simulink library "drivecyclelib"  (R2016a)
settings: Solver=ode45  StartTime=0.0  StopTime=10.0  RelTol=1e-3
undefined symbols (not defined in the file or in its folder): S_CYCLE, T_CYCLE, T_MAX
libraries: simulink x2
settings Model: Creator=e102261  LastModifiedBy=e102261
settings DataIOCC: LimitDataPoints=on  SaveFormat=Array
settings OptimizationCC: ExpressionDepthLimit=2147483647
settings DebuggingCC: UnderspecifiedInitializationDetection=Classic  MergeDetectMultiDrivingBlocksExec=none  SolverPrmCheckMsg=warning  MultiTaskDSMMsg=warning  MultiTaskCondExecSysMsg=none  FcnCallInpInsideContextMsg=EnableAllAsWarning  StateNameClashWarn=warning  StrictBusMsg=None
settings HardwareCC: ProdBitPerPointer=32  ProdLargestAtomicFloat=None  ProdIntDivRoundTo=Undefined  ProdEndianess=Unspecified  ProdWordSize=32  ProdHWDeviceType=32-bit Generic
settings ModelReferenceCC: PropagateSignalLabelsOutOfModel=off

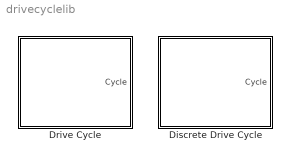
== system drivecyclelib ==
  Discrete Drive Cycle : Subsystem  mask(Discrete Drive Cycle){CycleName=NEDC, CycleRepeatsForever=off, SampleTime=0.1}
      mask prompts: CycleName "Cycle name:"; CycleRepeatsForever "Repeat cycle forever"; SampleTime "Sample time:"
      mask help: This block produces drive cycle data, as used in many automotive applications. It outputs displacement, velocity and acceleration, all in SI units. The user can choose from a list of popular cycles. Accuracy will suffer if the sample time gets too big: the maximum 'safe' value is one.
      mask init:
      | [S_CYCLE, T_CYCLE, T_MAX, W_SCALE, Disp, Vel, Acc, t, v] = ...
      |     drivecyclelib_maskInitFcn(CycleName, CycleRepeatsForever);
      mask TypeOptions CycleName: NEDC | ECE R15 | EUDC | ArtUrban | ArtRoad | ArtMw130 | ArtMw150 | WLTP class 3 | UDDS | FTP | HWFET
      mask Display:
      | color('yellow')
      | plot(t/max(t),3.6*v/160);
      | color('blue')
      | fprintf(CycleName);
  Drive Cycle : Subsystem  mask(Drive Cycle){CycleName=WLTP class 3, CycleRepeatsForever=off}
      mask prompts: CycleName "Cycle name:"; CycleRepeatsForever "Repeat cycle forever"
      mask help: This block produces drive cycle data, as used in many automotive applications. It outputs displacement, velocity and acceleration, all in SI units. The user can choose from a list of popular cycles.
      mask init:
      | [S_CYCLE, T_CYCLE, T_MAX, W_SCALE, Disp, Vel, Acc, t, v] = ...
      |     drivecyclelib_maskInitFcn(CycleName, CycleRepeatsForever);
      mask TypeOptions CycleName: NEDC | ECE R15 | EUDC | ArtUrban | ArtRoad | ArtMw130 | ArtMw150 | WLTP class 3 | UDDS | FTP | HWFET
      mask Display:
      | color('yellow')
      | plot(t/max(t),3.6*v/160);
      | color('blue')
      | fprintf(CycleName);

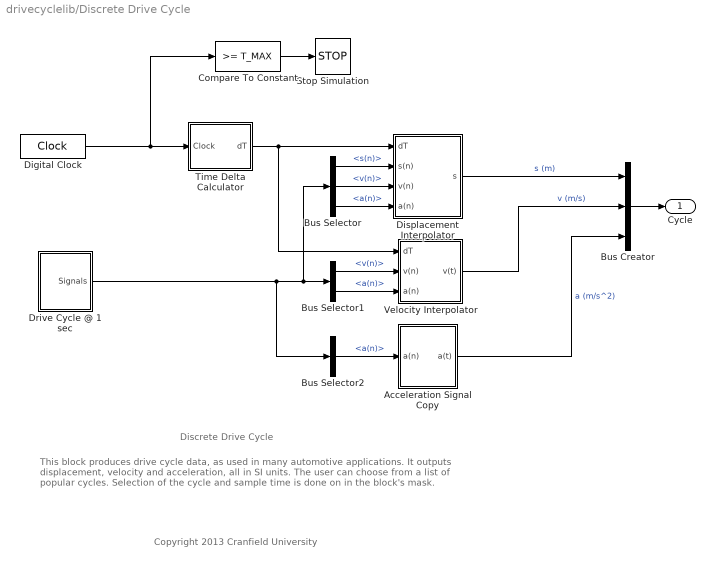
== system drivecyclelib/Discrete Drive Cycle ==
  note: This block produces drive cycle data, as used in many automotive applications.  It outputs
      | displacement, velocity and acceleration, all in SI units.  The user can choose from a list of
      | popular cycles.
      |
      | Selection of the cycle and sample time is done on in the block's mask.
  note: Copyright 2013 Cranfield University
  note: Discrete Drive Cycle
  Acceleration Signal Copy : Subsystem
  Bus Creator : BusCreator  Inputs=3
  Bus Selector : BusSelector  OutputSignals=s(n),v(n),a(n)
  Bus Selector1 : BusSelector  OutputSignals=v(n),a(n)
  Bus Selector2 : BusSelector  OutputSignals=a(n)
  Compare To Constant : simulink/Logic and Bit Operations/Compare To Constant  relop=>=  const=T_MAX  OutDataTypeStr=boolean
  Digital Clock : DigitalClock  SampleTime=SampleTime
  Displacement Interpolator : Subsystem
  Drive Cycle @ 1 sec : Subsystem
  Stop Simulation : Stop
  Time Delta Calculator : Subsystem
  Velocity Interpolator : Subsystem
  Cycle : Outport  SampleTime=SampleTime
  wires:
  Compare To Constant/1 -> Stop Simulation/1
  Time Delta Calculator/1(dT) -> Displacement Interpolator/1(dT), Velocity Interpolator/1(dT)
  Displacement Interpolator/1(s) -> Bus Creator/1  "s (m)"
  Velocity Interpolator/1(v(t)) -> Bus Creator/2  "v (m/s)"
  Drive Cycle @ 1 sec/1(Signals) -> Bus Selector/1, Bus Selector1/1, Bus Selector2/1
  Bus Selector/1 -> Displacement Interpolator/2(s(n))  "<s(n)>"
  Bus Selector/2 -> Displacement Interpolator/3(v(n))  "<v(n)>"
  Bus Selector/3 -> Displacement Interpolator/4(a(n))  "<a(n)>"
  Bus Selector1/1 -> Velocity Interpolator/2(v(n))  "<v(n)>"
  Bus Selector1/2 -> Velocity Interpolator/3(a(n))  "<a(n)>"
  Bus Selector2/1 -> Acceleration Signal Copy/1(a(n))  "<a(n)>"
  Acceleration Signal Copy/1(a(t)) -> Bus Creator/3  "a (m/s^2)"
  Bus Creator/1 -> Cycle/1
  Digital Clock/1 -> Time Delta Calculator/1(Clock), Compare To Constant/1

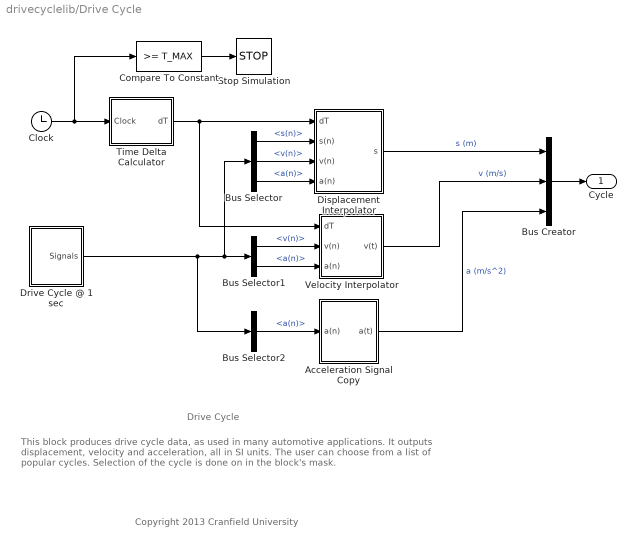
== system drivecyclelib/Drive Cycle ==
  note: This block produces drive cycle data, as used in many automotive applications.  It outputs
      | displacement, velocity and acceleration, all in SI units.  The user can choose from a list of
      | popular cycles.
      |
      | Selection of the cycle is done on in the block's mask.
  note: Copyright 2013 Cranfield University
  note: Drive Cycle
  Acceleration Signal Copy : Subsystem
  Bus Creator : BusCreator  Inputs=3
  Bus Selector : BusSelector  OutputSignals=s(n),v(n),a(n)
  Bus Selector1 : BusSelector  OutputSignals=v(n),a(n)
  Bus Selector2 : BusSelector  OutputSignals=a(n)
  Clock : Clock
  Compare To Constant : simulink/Logic and Bit Operations/Compare To Constant  relop=>=  const=T_MAX  OutDataTypeStr=boolean
  Displacement Interpolator : Subsystem
  Drive Cycle @ 1 sec : Subsystem
  Stop Simulation : Stop
  Time Delta Calculator : Subsystem
  Velocity Interpolator : Subsystem
  Cycle : Outport
  wires:
  Clock/1 -> Time Delta Calculator/1(Clock), Compare To Constant/1
  Bus Creator/1 -> Cycle/1
  Acceleration Signal Copy/1(a(t)) -> Bus Creator/3  "a (m/s^2)"
  Bus Selector2/1 -> Acceleration Signal Copy/1(a(n))  "<a(n)>"
  Bus Selector1/2 -> Velocity Interpolator/3(a(n))  "<a(n)>"
  Bus Selector1/1 -> Velocity Interpolator/2(v(n))  "<v(n)>"
  Bus Selector/3 -> Displacement Interpolator/4(a(n))  "<a(n)>"
  Bus Selector/2 -> Displacement Interpolator/3(v(n))  "<v(n)>"
  Bus Selector/1 -> Displacement Interpolator/2(s(n))  "<s(n)>"
  Drive Cycle @ 1 sec/1(Signals) -> Bus Selector2/1, Bus Selector1/1, Bus Selector/1
  Velocity Interpolator/1(v(t)) -> Bus Creator/2  "v (m/s)"
  Displacement Interpolator/1(s) -> Bus Creator/1  "s (m)"
  Time Delta Calculator/1(dT) -> Velocity Interpolator/1(dT), Displacement Interpolator/1(dT)
  Compare To Constant/1 -> Stop Simulation/1

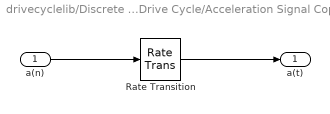
== system drivecyclelib/Discrete Drive Cycle/Acceleration Signal Copy ==
  a(n) : Inport
  Rate Transition : RateTransition  Integrity=off
  a(t) : Outport
  wires:
  a(n)/1 -> Rate Transition/1
  Rate Transition/1 -> a(t)/1

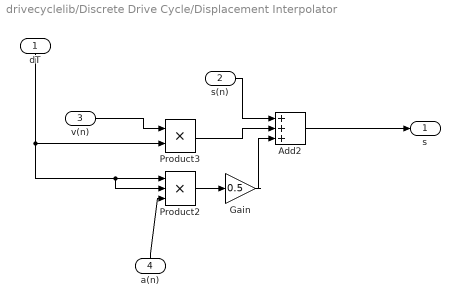
== system drivecyclelib/Discrete Drive Cycle/Displacement Interpolator ==
  dT : Inport
  s(n) : Inport  Port=2
  v(n) : Inport  Port=3
  a(n) : Inport  Port=4
  Add2 : Sum  Inputs=+++
  Gain : Gain  Gain=0.5
  Product2 : Product  Inputs=3  RndMeth=Zero
  Product3 : Product  RndMeth=Zero
  s : Outport
  wires:
  s(n)/1 -> Add2/1
  dT/1 -> Product3/2, Product2/2, Product2/1
  Product2/1 -> Gain/1
  Product3/1 -> Add2/2
  Add2/1 -> s/1
  Gain/1 -> Add2/3
  a(n)/1 -> Product2/3
  v(n)/1 -> Product3/1

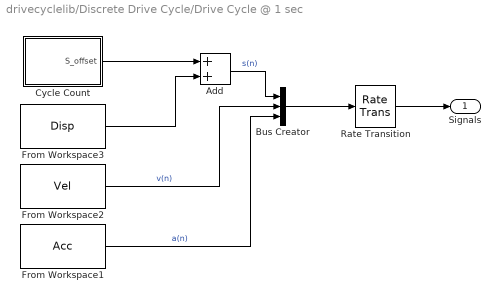
== system drivecyclelib/Discrete Drive Cycle/Drive Cycle @ 1 sec ==
  Add : Sum
  Bus Creator : BusCreator  Inputs=3
  Cycle Count : Subsystem
  From Workspace1 : FromWorkspace  VariableName=Acc  SampleTime=1  Interpolate=off  OutputAfterFinalValue=Cyclic repetition
  From Workspace2 : FromWorkspace  VariableName=Vel  SampleTime=1  Interpolate=off  OutputAfterFinalValue=Cyclic repetition
  From Workspace3 : FromWorkspace  VariableName=Disp  SampleTime=1  Interpolate=off  OutputAfterFinalValue=Cyclic repetition
  Rate Transition : RateTransition  Integrity=off  OutPortSampleTime=SampleTime
  Signals : Outport  SampleTime=SampleTime
  wires:
  Rate Transition/1 -> Signals/1
  Cycle Count/1(S_offset) -> Add/1
  From Workspace1/1 -> Bus Creator/3  "a(n)"
  From Workspace2/1 -> Bus Creator/2  "v(n)"
  From Workspace3/1 -> Add/2
  Add/1 -> Bus Creator/1  "s(n)"
  Bus Creator/1 -> Rate Transition/1

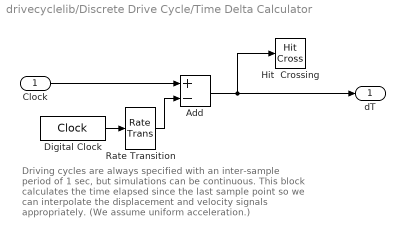
== system drivecyclelib/Discrete Drive Cycle/Time Delta Calculator ==
  note: Driving cycles are always specified with an inter-sample
      | period of 1 sec, but simulations can be continuous.  This
      | block calculates the time elapsed since the last sample
      | point so we can interpolate the displacement and velocity
      | signals appropriately.  (We assume uniform acceleration.)
  Clock : Inport
  Add : Sum  Inputs=+-
  Digital Clock : DigitalClock
  Hit  Crossing : HitCross  HitCrossingOffset=0.5  ShowOutputPort=off
  Rate Transition : RateTransition  Integrity=off  Deterministic=off  OutPortSampleTime=SampleTime
  dT : Outport
  wires:
  Digital Clock/1 -> Rate Transition/1
  Clock/1 -> Add/1
  Add/1 -> dT/1, Hit  Crossing/1
  Rate Transition/1 -> Add/2

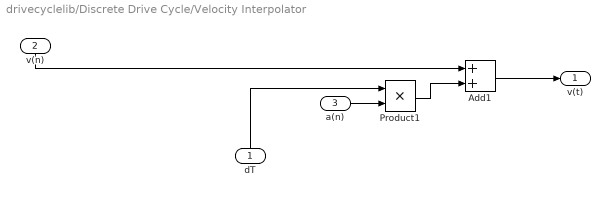
== system drivecyclelib/Discrete Drive Cycle/Velocity Interpolator ==
  dT : Inport
  v(n) : Inport  Port=2
  a(n) : Inport  Port=3
  Add1 : Sum
  Product1 : Product  RndMeth=Zero
  v(t) : Outport
  wires:
  Add1/1 -> v(t)/1
  a(n)/1 -> Product1/2
  v(n)/1 -> Add1/1
  dT/1 -> Product1/1
  Product1/1 -> Add1/2

== system drivecyclelib/Drive Cycle/Acceleration Signal Copy ==
  a(n) : Inport
  Rate Transition : RateTransition  Integrity=off
  a(t) : Outport
  wires:
  Rate Transition/1 -> a(t)/1
  a(n)/1 -> Rate Transition/1

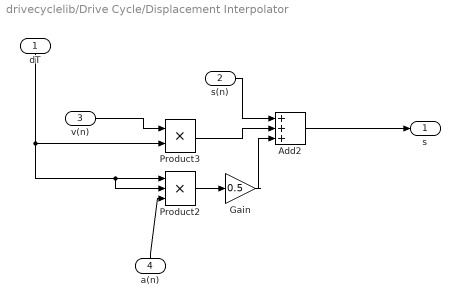
== system drivecyclelib/Drive Cycle/Displacement Interpolator ==
  dT : Inport
  s(n) : Inport  Port=2
  v(n) : Inport  Port=3
  a(n) : Inport  Port=4
  Add2 : Sum  Inputs=+++
  Gain : Gain  Gain=0.5
  Product2 : Product  Inputs=3  RndMeth=Zero
  Product3 : Product  RndMeth=Zero
  s : Outport
  wires:
  v(n)/1 -> Product3/1
  a(n)/1 -> Product2/3
  Gain/1 -> Add2/3
  Add2/1 -> s/1
  Product3/1 -> Add2/2
  Product2/1 -> Gain/1
  dT/1 -> Product2/1, Product2/2, Product3/2
  s(n)/1 -> Add2/1

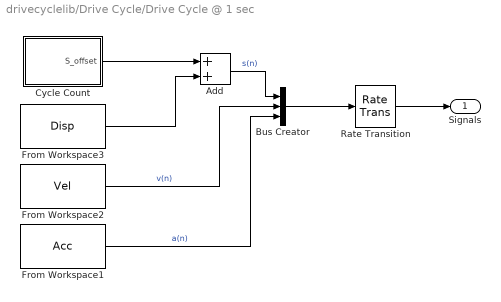
== system drivecyclelib/Drive Cycle/Drive Cycle @ 1 sec ==
  Add : Sum
  Bus Creator : BusCreator  Inputs=3
  Cycle Count : Subsystem
  From Workspace1 : FromWorkspace  VariableName=Acc  SampleTime=1  Interpolate=off  OutputAfterFinalValue=Cyclic repetition
  From Workspace2 : FromWorkspace  VariableName=Vel  SampleTime=1  Interpolate=off  OutputAfterFinalValue=Cyclic repetition
  From Workspace3 : FromWorkspace  VariableName=Disp  SampleTime=1  Interpolate=off  OutputAfterFinalValue=Cyclic repetition
  Rate Transition : RateTransition  Integrity=off  OutPortSampleTimeOpt=Inherit  OutPortSampleTime=SampleTime
  Signals : Outport  SampleTime=0
  wires:
  Rate Transition/1 -> Signals/1
  Cycle Count/1(S_offset) -> Add/1
  From Workspace1/1 -> Bus Creator/3  "a(n)"
  From Workspace2/1 -> Bus Creator/2  "v(n)"
  From Workspace3/1 -> Add/2
  Add/1 -> Bus Creator/1  "s(n)"
  Bus Creator/1 -> Rate Transition/1

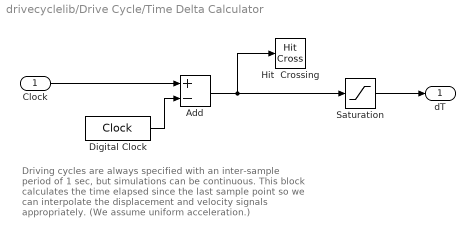
== system drivecyclelib/Drive Cycle/Time Delta Calculator ==
  note: Driving cycles are always specified with an inter-sample
      | period of 1 sec, but simulations can be continuous.  This
      | block calculates the time elapsed since the last sample
      | point so we can interpolate the displacement and velocity
      | signals appropriately.  (We assume uniform acceleration.)
  Clock : Inport
  Add : Sum  Inputs=+-
  Digital Clock : DigitalClock
  Hit  Crossing : HitCross  HitCrossingOffset=0.5  HitCrossingDirection=falling  ShowOutputPort=off
  Saturation : Saturate  UpperLimit=1  LowerLimit=0  ZeroCross=off
  dT : Outport
  wires:
  Saturation/1 -> dT/1
  Add/1 -> Hit  Crossing/1, Saturation/1
  Clock/1 -> Add/1
  Digital Clock/1 -> Add/2

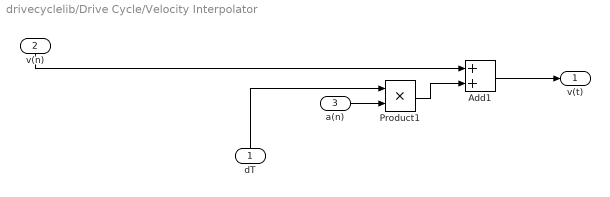
== system drivecyclelib/Drive Cycle/Velocity Interpolator ==
  dT : Inport
  v(n) : Inport  Port=2
  a(n) : Inport  Port=3
  Add1 : Sum
  Product1 : Product  RndMeth=Zero
  v(t) : Outport
  wires:
  Product1/1 -> Add1/2
  dT/1 -> Product1/1
  v(n)/1 -> Add1/1
  a(n)/1 -> Product1/2
  Add1/1 -> v(t)/1

== system drivecyclelib/Discrete Drive Cycle/Drive Cycle @ 1 sec/Cycle Count ==
  MATLAB Function : MATLAB Function  TreatAsAtomicUnit=on
  S_offset : Outport
  wires:
  MATLAB Function/1(S_offset) -> S_offset/1

== system drivecyclelib/Drive Cycle/Drive Cycle @ 1 sec/Cycle Count ==
  MATLAB Function : MATLAB Function  TreatAsAtomicUnit=on
  S_offset : Outport
  wires:
  MATLAB Function/1(S_offset) -> S_offset/1

== matlab function drivecyclelib/Discrete Drive Cycle/Drive Cycle @ 1 sec/Cycle Count/MATLAB Function ==
  settings: updateMethod=DISCRETE  sampleTime=1
  data: S_offset output; T_CYCLE parameter; S_CYCLE parameter
function S_offset = calcDispOffset(T_CYCLE, S_CYCLE)
%#codegen

persistent sampleCount cycleCount T_CYCLE_uint32;
if isempty(cycleCount)    
    sampleCount = uint32(0);
    cycleCount  = uint32(0);
    T_CYCLE_uint32 = uint32(T_CYCLE);
end

while sampleCount >= T_CYCLE_uint32;
    cycleCount = cycleCount + uint32(1);
    sampleCount = sampleCount - T_CYCLE_uint32;
end

S_offset = S_CYCLE * double(cycleCount);

sampleCount = sampleCount + uint32(1);
end

== matlab function drivecyclelib/Drive Cycle/Drive Cycle @ 1 sec/Cycle Count/MATLAB Function ==
  settings: updateMethod=DISCRETE  sampleTime=1
  data: S_offset output; T_CYCLE parameter; S_CYCLE parameter
function S_offset = calcDispOffset(T_CYCLE, S_CYCLE)
%#codegen

persistent sampleCount cycleCount T_CYCLE_uint32;
if isempty(cycleCount)    
    sampleCount = uint32(0);
    cycleCount  = uint32(0);
    T_CYCLE_uint32 = uint32(T_CYCLE);
end

while sampleCount >= T_CYCLE_uint32;
    cycleCount = cycleCount + uint32(1);
    sampleCount = sampleCount - T_CYCLE_uint32;
end

S_offset = S_CYCLE * double(cycleCount);

sampleCount = sampleCount + uint32(1);
end
